simulink model "WMMSupportingForcesGP2021b"  (R2021b)
settings: Solver=ode23t  StartTime=0.0  StopTime=inf  FixedStep=.001  RelTol=1e-3  AbsTol=1e-3
InitFcn:
  | InitializeSimulationGP
  | SimulationParametersGP
values from neighbouring files (symbols this model uses):
  B11_r_B11C = [0.23805608; 0.13201777; 0]    [InitializeSimulationGP.m]
  B11_r_B11Tc1 = [L11; 0; 0]    [InitializeSimulationGP.m]
  B11_Rot_Tc1 = eye(3)    [InitializeSimulationGP.m]
  B11cI = [0.28426000 -0.06487287 0;         -0.06487287  0.54237481 0;                   0  0          0.67891020]    [InitializeSimulationGP.m]
  B12_r_B12C = [0.60504569; 0.27199376; 0.00002484]    [InitializeSimulationGP.m]
  B12_r_B12Tc2 = [L12;0;0]    [InitializeSimulationGP.m]
  B12_Rot_Tc2 = eye(3)    [InitializeSimulationGP.m]
  B12cI = [1.18803886 -2.36786418 0.00280315;          -2.36786418 6.31493281 0.00022322;           0.00280315 0.00022322 7.40915161]    [InitializeSimulationGP.m]
  B31_r_B31C = [0.35781210 0 0]    [InitializeSimulationGP.m]
  B31_Rot_B41 = eye(3)    [InitializeSimulationGP.m]
  B31cI = diag([0.03150902 0.90735702 0.90763033])    [InitializeSimulationGP.m]
  B32_r_B32C = [0.35781210 0 0]    [InitializeSimulationGP.m]
  B32_Rot_B42 = eye(3)    [InitializeSimulationGP.m]
  B32cI = diag([0.03150902 0.90735702 0.90763033])    [InitializeSimulationGP.m]
  B41_r_B41C = [0.55785997 0 0]    [InitializeSimulationGP.m]
  B41_r_B41Tc1 = [lc1;0;0]    [InitializeSimulationGP.m]
  B41cI = diag([0.00370720 0.55759812 0.55785997])    [InitializeSimulationGP.m]
  B42_r_B42C = [0.55785997 0 0]    [InitializeSimulationGP.m]
  B42_r_B42Tc2 = [lc2; 0; 0]    [InitializeSimulationGP.m]
  B42cI = diag([0.00370720 0.55759812 0.55785997])    [InitializeSimulationGP.m]
  B52_r_B52C = [0 0 0.56802906]    [InitializeSimulationGP.m]
  B52_r_B52P32 = [lc3; 0; 0]    [InitializeSimulationGP.m]
  B52_Rot_P32 = eye(3)    [InitializeSimulationGP.m]
  B52cI = diag([0.91789884, 0.91790043, 0.00091463])    [InitializeSimulationGP.m]
  Bc1_r_Bc1B11 = [L1; 0; 0]    [InitializeSimulationGP.m]
  Bc1_r_Bc1B31 = [0;0;0]    [InitializeSimulationGP.m]
  Bc1_r_Bc1C = [0.14178771; 0.16555780; 0]    [InitializeSimulationGP.m]
  Bc1_V = [0;0;0;0;0;0]    [InitializeSimulationGP.m]
  Bc1cI = [+5.892211080 +5.476111360 -0.000019630;          +5.476111360 +28.66965601 -0.000024550;          -0.000019630 -0.000024550 +29.78955950]    [InitializeSimulationGP.m]
  Bc2_r_Bc2B12 = [L2;0;0]    [InitializeSimulationGP.m]
  Bc2_r_Bc2B32 = [0;0;0]    [InitializeSimulationGP.m]
  Bc2_r_Bc2C = [0.54319901; 0.10543875; 0]    [InitializeSimulationGP.m]
  Bc2cI = [0.48071390 0.52924041 0;          0.52924041 5.80912352 0;              0      0          5.97255351]    [InitializeSimulationGP.m]
  BC_r_BCBM = [xCA; yCA; zCA]    [SimulationParametersGP.m]
  BC_Rot_BM = eye(3)    [SimulationParametersGP.m]
  BCI = diag([100 1200 1000])    [SimulationParametersGP.m]
  beta1 = atan2d(374.261,935)*pi/180    [InitializeSimulationGP.m]
  beta2 = atan2d(45.757,373.313)*pi/180    [InitializeSimulationGP.m]
  beta3 = atan2d(139.50,1132.19)*pi/180    [InitializeSimulationGP.m]
  beta4 = atan2d(88.061,296.198)*pi/180    [InitializeSimulationGP.m]
  betaGround = 1e6    (= 1000000)    [SimulationParametersGP.m]
  BFL = 0.05    [SimulationParametersGP.m]
  BFR = 0.05    [SimulationParametersGP.m]
  BM_r_BMBMp = [0;0;0]    [SimulationParametersGP.m]
  BM_Rot_BMp = [cos(gamma) -sin(gamma) 0; sin(gamma) cos(gamma) 0; 0 0 1]    [SimulationParametersGP.m]
  BMp_r_BMpBc1 = [0.185;0;0.205]    [InitializeSimulationGP.m]
  BMp_Rot_Bc1 = [cos(alpha1) -sin(alpha1)  0;                  0            0       -1;                sin(alpha1)  cos(alpha1)  0]    [InitializeSimulationGP.m]
  BRL = 0.05    [SimulationParametersGP.m]
  BRR = 0.05    [SimulationParametersGP.m]
  cc = 0.0    (= 0)    [SimulationParametersGP.m]
  D22F = [0;0;0;0;0;0]    [InitializeSimulationGP.m]
  dT = 0.01    [SimulationParametersGP.m]
  g0 = 9.8066    [SimulationParametersGP.m]
  ground_stiffness = 1e8    (= 100000000)    [SimulationParametersGP.m]
  l1 = 1.15-cc    (= 1.15)    [SimulationParametersGP.m]
  L1 = 1.0071227324212    (= 1.00712273242)    [InitializeSimulationGP.m]
  L11 = 0.37610632101293    (= 0.376106321013)    [InitializeSimulationGP.m]
  L12 = 0.30901132665325    (= 0.309011326653)    [InitializeSimulationGP.m]
  l2 = 1.15+cc    (= 1.15)    [SimulationParametersGP.m]
  L2 = 1.132185817991    (= 1.13218581799)    [InitializeSimulationGP.m]
  lc1 = 0.745    [InitializeSimulationGP.m]
  lc2 = 0.745    [InitializeSimulationGP.m]
  mB11 = 25.52660174    [InitializeSimulationGP.m]
  mB12 = 33.92850233    [InitializeSimulationGP.m]
  mB31 = 17.36281648    [InitializeSimulationGP.m]
  mB32 = 17.36281648    [InitializeSimulationGP.m]
  mB41 = 10.34519231    [InitializeSimulationGP.m]
  mB42 = 10.34519231    [InitializeSimulationGP.m]
  mB52 = 6.73059863    [InitializeSimulationGP.m]
  mBC = 2200    [SimulationParametersGP.m]
  mBc1 = 307.29601379    [InitializeSimulationGP.m]
  mBc2 = 54.58702836    [InitializeSimulationGP.m]
  mFL = 60    [SimulationParametersGP.m]
  mFR = 60    [SimulationParametersGP.m]
  mP22 = 9.26136143    [InitializeSimulationGP.m]
  mP32 = 570.18877059    [InitializeSimulationGP.m]
  mRR = 60    [SimulationParametersGP.m]
  mw = mFL    (= 60)    [SimulationParametersGP.m]
  P22_r_P22C = [0.62192523 0 0]    [InitializeSimulationGP.m]
  P22_Rot_B52 = eye(3)    [InitializeSimulationGP.m]
  P22cI = diag([0.00662754, 1.48387017, 1.48398069])    [InitializeSimulationGP.m]
  P32_r_P32C = [0.25466704; -0.13034397; -0.01302248]    [InitializeSimulationGP.m]
  P32_r_P32D22 = [0.40499744871392; -0.13130517281345; -0.013385243295654]    [InitializeSimulationGP.m]
  P32_Rot_D22 = [1 0 0;              0 0.9707729441837 0.23999977258512;              0 -0.23999977258512 0.9707729441837]    [InitializeSimulationGP.m]
  P32cI = [46.81220713 0.38607676 -0.00453819;          0.38607676 71.92201786 -1.14320993;          -0.00453819 -1.14320993 67.38128576]    [InitializeSimulationGP.m]
  R0FL = 0.35    [SimulationParametersGP.m]
  R0FR = 0.35    [SimulationParametersGP.m]
  R0RL = 0.35    [SimulationParametersGP.m]
  R0RR = 0.35    [SimulationParametersGP.m]
  Rw = R0FL    (= 0.35)    [SimulationParametersGP.m]
  Tc1_r_Tc1Bc2 = [0.098495302558553; 0.01838181329939; 0]    [InitializeSimulationGP.m]
  Tc1_Rot_Bc2 = [cos(alpha2) -sin(alpha2) 0;                sin(alpha2)  cos(alpha2) 0;                0            0           1]    [InitializeSimulationGP.m]
  Tc2_r_Tc2P22 = [-0.048858374920227;0.36587359346146;0.035276938723102]    [InitializeSimulationGP.m]
  Tc2_Rot_P22 = [0.95853460763586 -0.27664713597974  0.0683942111482;                0.28497614981675  0.93051946315663 -0.23004808784757;                0                 0.23999977258511  0.9707729441837]    [InitializeSimulationGP.m]
  Th1A = 10*pi/180    (= 0.174532925199)    [InitializeSimulationGP.m]
  Th1B = 20*pi/180    (= 0.349065850399)    [InitializeSimulationGP.m]
  Th1f = 1    [InitializeSimulationGP.m]
  Th2A = 15*pi/180    (= 0.261799387799)    [InitializeSimulationGP.m]
  Th2B = -70*pi/180    (= -1.2217304764)    [InitializeSimulationGP.m]
  Th2f = 2    [InitializeSimulationGP.m]
  w = wFL    (= 0.875)    [SimulationParametersGP.m]
  W_r_WBc1 = [0.185;0;0.205]    [InitializeSimulationGP.m]
  W_Rot_Bc1 = [cos(alpha1) -sin(alpha1)  0;                  0            0       -1;                sin(alpha1)  cos(alpha1)  0]    [InitializeSimulationGP.m]
  x10 = 0.83    [InitializeSimulationGP.m]
  x20 = 0.83    [InitializeSimulationGP.m]
  x3A = 0.2    [InitializeSimulationGP.m]
  x3B = 0.3    [InitializeSimulationGP.m]
  x3f = 1    [InitializeSimulationGP.m]
  xCA = 0.5    [SimulationParametersGP.m]
  xf = [1;0;0;0;0;0]    [InitializeSimulationGP.m]
  yCA = 0    [SimulationParametersGP.m]
  zC = 0.45    [SimulationParametersGP.m]
  zCA = .25    (= 0.25)    [SimulationParametersGP.m]
  ztau = [0;0;0;0;0;1]    [InitializeSimulationGP.m]
undefined symbols (not defined in the file or in its folder): alphaFL_meas, alphaFR_meas, alphaRL_meas, alphaRR_meas, B11_V, B11Ftot, B12_U_Tc2, B12_V, B12Ftot, B31_r_B31B41, B31_V, B31FTot, B32_r_B32B42, B32_U_B42, B32_V, B32FTot, B41_V, B41FTot, B42_Rot_Tc2, B42_U_Tc2, B42_V, B42FTot, B52_U_P32, B52_V, B52Ftot, Bc1Tot, Bc2_Rot_B12, Bc2_Rot_B32, Bc2_U_B12, Bc2_U_B32, Bc2_V, Bc2Tot, betaC_meas, D22_V, deltaFL_cmd, deltaFL_meas, deltaFR_cmd, deltaFR_meas, deltaRL_cmd, deltaRL_meas, deltaRR_cmd, deltaRR_meas, dOmegaFL_meas, dOmegaFR_meas, dOmegaRL_meas, dOmegaRR_meas, dPsi_meas, dq1, dq11, dq12, dq2, dq21, dq22, dx1, dx2, Floor, FTot_S1, FTot_S2P, FTot_S2R, FzFL ... (+63)
libraries: sm_lib x94, nesl_utility x63, simulink x5
(part 1 of 11)
settings Model: SimulationMode=accelerator  Creator=pvgope  LastModifiedBy=pvgope
settings SolverCC: InitialStep=.0001  ZeroCrossAlgorithm=Adaptive
settings DebuggingCC: IgnoredZcDiagnostic=none
settings DiagnosticsConfigSet: SimMechanicsRigidlyBoundBlock=warning
settings ExplorerConfigSet: InternalSimMechanicsExplorerSettings="<ExplorerConfiguration><canonicalview>default</canonicalview><AnimationSetting><BasePlaybackSpeed>1.0</BasePlaybackSpeed><PlaybackSpeedFactor>2.0</PlaybackSpeedFactor></AnimationSetting><TilePanel><TileInfo><Tiles Columns=\"1\" Count=\"1\" Rows=\"1\"><Column Weight=\"1\"/><Row Weight=\"1\"/><Tile Height=\"1\" Width=\"1\" X=\"0\" Y=\"0\"/></Tiles></TileInfo><SceneInfo><SceneViewer><BGColor><R>0.60000002384185791</R><G>0.60000002384185791</G><B>0.60000002384185791</B></BGColor><Camera><DoPerspective>on</DoPerspective><Position><X>510.5</X><Y>-7.37257477290143015e-18</Y><Z>5.70000000000000195</Z></Position><Center><X>509.560307379214066</X><Y>-7.22248032388580699e-18</Y><Z>5.35797985667433352</Z></Center><Up><X>-0.342020143325668713</X><Y>-4.59743080112967589e-18</Y><Z>0.939692620785908428</Z></Up><ViewLimDist>1</ViewLimDist><YLim>0.466307658154998583</YLim><XLim>0.717896906275835023</XLim></Camera></SceneViewer></SceneInfo></TilePanel><MechEditorPanel><Cameras><Camera><Id>Camera1</Id><Value><Name>Camera1</Name><NativeCamera><PositionTrackingFeature>Mobile_Manipulator_in_Simscape.Camera0.R</PositionTrackingFeature><CenterTrackingFeature>Mobile_Manipulator_in_Simscape.Camera0.R</CenterTrackingFeature><UpVectorTrackingFeature>Mobile_Manipulator_in_Simscape.Camera0.R</UpVectorTrackingFeature><CenterTrackingOrigin>off</CenterTrackingOrigin><CenterTrackingDirection>-X</CenterTrackingDirection><UpVectorTrackingDirection>+Z</UpVectorTrackingDirection></NativeCamera></Value></Camera></Cameras><GfxPanelCameraMap><MapElement CameraMLId=\"Camera1\" GfxPanelIndex=\"0\"/></GfxPanelCameraMap><VideoCreator><PlaybackSpeedRatio>2.0</PlaybackSpeedRatio><FrameRate>60</FrameRate><VideoFormat>Motion JPEG AVI</VideoFormat><FrameSize>[1280 720]</FrameSize></VideoCreator></MechEditorPanel></ExplorerConfiguration>"

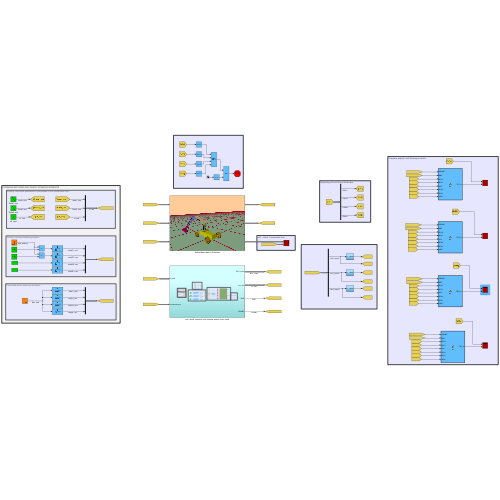
[thumbnail: Simulink's stored preview of the top-level diagram]
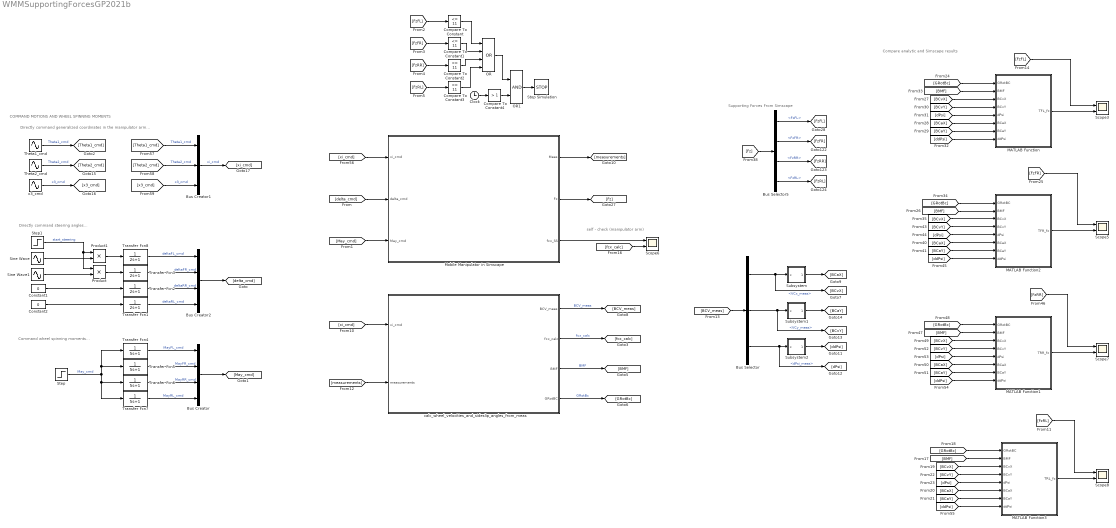
== system WMMSupportingForcesGP2021b ==
  note: Compare analytic and Simscape results
  note: Supporting Forces From Simscape
  note: COMMAND MOTIONS AND WHEEL SPINNING MOMENTS
  note: self - check (manipulator arm)
  note: Directly command generalized coordinates in the manipulator arm...
  note: Directly command steering angles...
  note: Command wheel spinning moments...
  Bus Creator : BusCreator  Inputs=MayFL_cmd,MayFR_cmd,MayRR_cmd,MayRL_cmd
  Bus Creator1 : BusCreator  Inputs=3
  Bus Creator2 : BusCreator  Inputs=deltaFL_cmd,deltaFR_cmd,deltaRR_cmd,deltaRL_cmd
  Bus Selector : BusSelector  OutputSignals=VCx_meas,VCy_meas,dPsi_meas
  Bus Selector5 : BusSelector  OutputSignals=FzFL,FzFR,FzRR,FzRL
  Clock : Clock
  Compare To Constant{,1..3} (4 alike) : simulink/Logic and Bit Operations/Compare To Constant  relop=<=  const=11  OutDataTypeStr=boolean
  Compare To Constant4 : simulink/Logic and Bit Operations/Compare To Constant  relop=>  const=1  OutDataTypeStr=boolean
  Constant1 : Constant  Value=0
  Constant2 : Constant  Value=0
  MATLAB Function : MATLAB Function  TreatAsAtomicUnit=on
  MATLAB Function1 : MATLAB Function  TreatAsAtomicUnit=on
  MATLAB Function2 : MATLAB Function  TreatAsAtomicUnit=on
  MATLAB Function3 : MATLAB Function  TreatAsAtomicUnit=on
  Mobile Manipulator in Simscape : Subsystem
      mask Display: image('$imagefile'); % Use "Edit Image" on toolstrip to change.
  OR : Logic  Operator=OR  Inputs=4  AllPortsSameDT=off  OutDataTypeStr=boolean
  OR1 : Logic  AllPortsSameDT=off  OutDataTypeStr=boolean
  Product : Product
  Product1 : Product
  Scope{3,5..8} (5 alike) : Scope  NumInputPorts=2
  Sine Wave : Sin  Amplitude=4*pi/180  Frequency=.9  SampleTime=0
  Sine Wave1 : Sin  Amplitude=4*pi/180  Frequency=.9  SampleTime=0
  Step : Step  Time=15  Before=50  After=-50  SampleTime=0
  Step1 : Step  Time=30  SampleTime=0
  Stop Simulation : Stop
  Subsystem : Subsystem
  Subsystem1 : Subsystem
  Subsystem2 : Subsystem
  Theta1_cmd : Sin  Amplitude=Th1A  Bias=Th1B  Frequency=Th1f  SampleTime=0
  Theta2_cmd : Sin  Amplitude=Th2A  Bias=Th2B  Frequency=Th2f  SampleTime=0
  Transfer Fcn{1..3,8} (4 alike) : TransferFcn  Denominator=[2 1]
  Transfer Fcn{4..7} (4 alike) : TransferFcn  Denominator=[5 1]
  calc_wheel_velocities_and_sideslip_angles_from_meas : Subsystem
  x3_cmd : Sin  Amplitude=x3A  Bias=x3B  Frequency=x3f  SampleTime=0
  wires:
  [delta_cmd] -> Mobile Manipulator in Simscape/2(delta_cmd)
  Bus Creator2/1 -> [delta_cmd]
  Transfer Fcn8/1 -> Bus Creator2/1  "deltaFL_cmd"
  Transfer Fcn3/1 -> Bus Creator2/2  "deltaFR_cmd"
  Transfer Fcn2/1 -> Bus Creator2/3  "deltaRR_cmd"
  Transfer Fcn1/1 -> Bus Creator2/4  "deltaRL_cmd"
  [May_cmd] -> Mobile Manipulator in Simscape/3(May_cmd)
  Mobile Manipulator in Simscape/1(Meas) -> [measurements]
  [measurements] -> calc_wheel_velocities_and_sideslip_angles_from_meas/2(measurements)
  calc_wheel_velocities_and_sideslip_angles_from_meas/1(BCV_meas) -> [BCV_meas]  "BCV_meas"
  Constant1/1 -> Transfer Fcn2/1
  Mobile Manipulator in Simscape/2(Fz) -> [Fz]
  [Fz] -> Bus Selector5/1
  Bus Selector5/1 -> [FzFL]  "<FzFL>"
  Bus Selector5/2 -> [FzFR]  "<FzFR>"
  Bus Selector5/3 -> [FzRR]  "<FzRR>"
  Bus Selector5/4 -> [FzRL]  "<FzRL>"
  Bus Creator/1 -> [May_cmd]
  Constant2/1 -> Transfer Fcn1/1
  calc_wheel_velocities_and_sideslip_angles_from_meas/2(fcx_calc) -> [fcx_calc]  "fcx_calc"
  [fcx_calc] -> Scope6/2
  calc_wheel_velocities_and_sideslip_angles_from_meas/4(GRotBC) -> [GRotBc]  "GRotBc"
  [BCV_meas] -> Bus Selector/1
  Subsystem/1(dx/dt) -> [BCaX]
  Bus Selector/1 -> [BCvX], Subsystem/1(x)  "<VCx_meas>"
  Bus Selector/2 -> [BCvY], Subsystem1/1(x)  "<VCy_meas>"
  Bus Selector/3 -> [dPsi], Subsystem2/1(x)  "<dPsi_meas>"
  Subsystem2/1(dx/dt) -> [ddPsi]
  Subsystem1/1(dx/dt) -> [BCaY]
  Transfer Fcn4/1 -> Bus Creator/1  "MayFL_cmd"
  Transfer Fcn5/1 -> Bus Creator/2  "MayFR_cmd"
  Transfer Fcn6/1 -> Bus Creator/3  "MayRR_cmd"
  Transfer Fcn7/1 -> Bus Creator/4  "MayRL_cmd"
  [GRotBc] -> MATLAB Function/1(GRotBC)
  [ddPsi] -> MATLAB Function1/8(ddPsi)
  [BMF] -> MATLAB Function1/2(BMF)
  [BCvX] -> MATLAB Function2/3(BCvX)
  [FzFR] -> Scope5/1
  [BCaX] -> MATLAB Function/6(BCaX)
  [BCvX] -> MATLAB Function/3(BCvX)
  [BCvX] -> MATLAB Function1/3(BCvX)
  [BCvY] -> MATLAB Function1/4(BCvY)
  [BCaX] -> MATLAB Function1/6(BCaX)
  [FzFL] -> Scope3/1
  [ddPsi] -> MATLAB Function2/8(ddPsi)
  MATLAB Function/1(TFL_fz) -> Scope3/2
  [BCaY] -> MATLAB Function2/7(BCaY)
  [BCaX] -> MATLAB Function2/6(BCaX)
  [GRotBc] -> MATLAB Function2/1(GRotBC)
  [BCvY] -> MATLAB Function2/4(BCvY)
  [BCvY] -> MATLAB Function/4(BCvY)
  [BMF] -> MATLAB Function/2(BMF)
  MATLAB Function2/1(TFR_fz) -> Scope5/2
  [BMF] -> MATLAB Function2/2(BMF)
  [ddPsi] -> MATLAB Function/8(ddPsi)
  [GRotBc] -> MATLAB Function1/1(GRotBC)
  MATLAB Function1/1(TRR_fz) -> Scope7/2
  [dPsi] -> MATLAB Function/5(dPsi)
  [BCaY] -> MATLAB Function1/7(BCaY)
  [FzRR] -> Scope7/1
  [dPsi] -> MATLAB Function1/5(dPsi)
  [BCaY] -> MATLAB Function/7(BCaY)
  [dPsi] -> MATLAB Function2/5(dPsi)
  [dPsi] -> MATLAB Function3/5(dPsi)
  [FzRL] -> Scope8/1
  [BCaY] -> MATLAB Function3/7(BCaY)
  [GRotBc] -> MATLAB Function3/1(GRotBC)
  [BCaX] -> MATLAB Function3/6(BCaX)
  [BCvY] -> MATLAB Function3/4(BCvY)
  [BCvX] -> MATLAB Function3/3(BCvX)
  [BMF] -> MATLAB Function3/2(BMF)
  [ddPsi] -> MATLAB Function3/8(ddPsi)
  Sine Wave1/1 -> Product/2
  Product/1 -> Transfer Fcn3/1
  Product1/1 -> Transfer Fcn8/1
  Sine Wave/1 -> Product1/2
  Step1/1 -> Product/1, Product1/1  "start_steering"
  MATLAB Function3/1(TRL_fz) -> Scope8/2
  calc_wheel_velocities_and_sideslip_angles_from_meas/3(BMF) -> [BMF]  "BMF"
  Theta1_cmd/1 -> [Theta1_cmd]  "Theta1_cmd"
  Theta2_cmd/1 -> [Theta2_cmd]  "Theta2_cmd"
  x3_cmd/1 -> [x3_cmd]  "x3_cmd"
  [xi_cmd] -> Mobile Manipulator in Simscape/1(xi_cmd)
  [x3_cmd] -> Bus Creator1/3  "x3_cmd"
  [Theta2_cmd] -> Bus Creator1/2  "Theta2_cmd"
  [Theta1_cmd] -> Bus Creator1/1  "Theta1_cmd"
  Bus Creator1/1 -> [xi_cmd]  "xi_cmd"
  Step/1 -> Transfer Fcn5/1, Transfer Fcn4/1, Transfer Fcn7/1, Transfer Fcn6/1  "May_cmd"
  Mobile Manipulator in Simscape/3(fcx_SS) -> Scope6/1
  [xi_cmd] -> calc_wheel_velocities_and_sideslip_angles_from_meas/1(xi_cmd)
  Compare To Constant1/1 -> OR/2
  OR/1 -> OR1/1
  Clock/1 -> Compare To Constant4/1
  Compare To Constant4/1 -> OR1/2
  [FzFR] -> Compare To Constant1/1
  Compare To Constant2/1 -> OR/3
  OR1/1 -> Stop Simulation/1
  [FzFL] -> Compare To Constant/1
  Compare To Constant/1 -> OR/1
  [FzRL] -> Compare To Constant3/1
  Compare To Constant3/1 -> OR/4
  [FzRR] -> Compare To Constant2/1
